simulink model "EKF2nd_order_4_parameters_simulink"  (R2022a)
settings: Solver=ode1  StartTime=0.0  StopTime=10  FixedStep=0.01  RelTol=1e-3
settings Model: Creator=Sarot PC  LastModifiedBy=LabPC
settings SolverCC: AlgebraicLoopSolver=TrustRegion
settings DebuggingCC: UnconnectedInputMsg=warning  UnconnectedOutputMsg=warning  UnconnectedLineMsg=warning  SFMachineParentedDataDiag=warning
settings RTWCC: DLArmComputeVersion=19.05

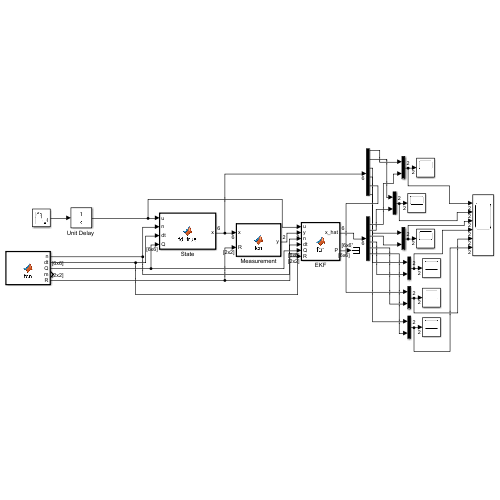
[thumbnail: Simulink's stored preview of the top-level diagram]
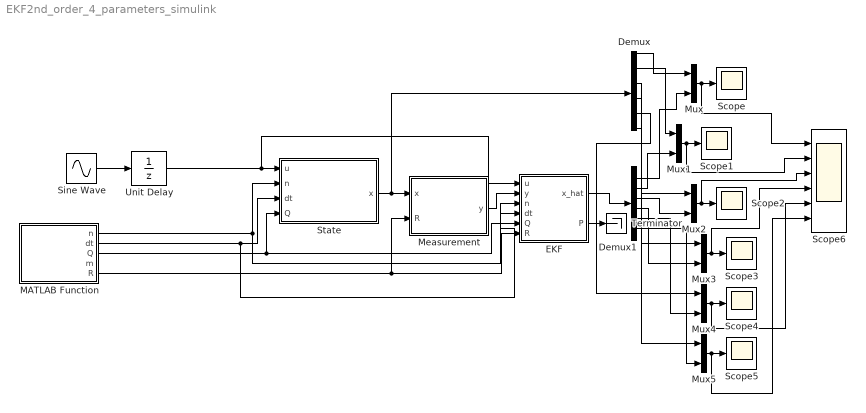
== system EKF2nd_order_4_parameters_simulink ==
  Demux : Demux  Outputs=6
  Demux1 : Demux  Outputs=6
  EKF : MATLAB Function  TreatAsAtomicUnit=on
  MATLAB Function : MATLAB Function  TreatAsAtomicUnit=on
  Measurement : MATLAB Function  TreatAsAtomicUnit=on
  Mux{,1..5} (6 alike) : Mux  Inputs=2
  Scope{,1..5} (6 alike) : Scope
  Scope6 : Scope  NumInputPorts=6
  Sine Wave : Sin  Amplitude=10  Frequency=2*pi*1.1
  State : MATLAB Function  TreatAsAtomicUnit=on
  Terminator : Terminator
  "Unit Delay " : UnitDelay  SampleTime=-1  HasFrameUpgradeWarning=on
  wires:
  State/1(x) -> Demux/1, Measurement/1(x)
  Measurement/1(y) -> EKF/2(y)
  EKF/1(x_hat) -> Demux1/1
  EKF/2(P) -> Terminator/1
  Demux/1 -> Mux/1
  Demux1/1 -> Mux/2
  Demux/2 -> Mux1/1
  Mux/1 -> Scope6/1, Scope/1
  Demux1/2 -> Mux1/2
  Demux/3 -> Mux2/1
  Demux1/3 -> Mux2/2
  Mux1/1 -> Scope6/2, Scope1/1
  Mux2/1 -> Scope6/3, Scope2/1
  Sine Wave/1 -> "Unit Delay "/1
  "Unit Delay "/1 -> EKF/1(u), State/1(u)
  MATLAB Function/1(n) -> EKF/3(n), State/2(n)
  MATLAB Function/2(dt) -> EKF/4(dt), State/3(dt)
  MATLAB Function/3(Q) -> EKF/5(Q), State/4(Q)
  MATLAB Function/5(R) -> EKF/6(R), Measurement/2(R)
  Mux3/1 -> Scope6/4, Scope3/1
  Demux/4 -> Mux3/1
  Demux1/4 -> Mux3/2
  Demux/5 -> Mux4/1
  Mux4/1 -> Scope6/5, Scope4/1
  Mux5/1 -> Scope6/6, Scope5/1
  Demux/6 -> Mux5/1
  Demux1/5 -> Mux4/2
  Demux1/6 -> Mux5/2

== matlab function EKF2nd_order_4_parameters_simulink/State ==
  settings: updateMethod=DISCRETE
  data: u input; x output; n input; dt input; Q input
function x = fd_true(u,n,dt,Q)

persistent x_
if isempty(x_),x_ = [0;0;10;20;40;30];end

% omega_ddot = -a*omega - b*omega_dot + c*u - d*sign(omega)
% Let x1=omega, x2=omega_dot, x3=a, x4=b, x5=c, x6=d
% x1_dot=-x2
% x2_dot=-x3*x1-x4*x2+x5*u-x6*sign(x1)
% x3_dot=0
% x4_dot=0
% x5_dot=0
% x6_dot=0

x = [x_(1) + dt*x_(2)
     x_(2) + dt*(-x_(3)*x_(1) - x_(4)*x_(2) + x_(5)*u - x_(6)*sign(x_(1)))
     x_(3)
     x_(4)
     x_(5)
     x_(6)] + sqrt(dt)*sqrt(Q)*randn(n,1);
x_= x;

== matlab function EKF2nd_order_4_parameters_simulink/MATLAB Function ==
  data: n output; dt output; Q output; m output; R output
function [n,dt,Q,m,R] = fcn

n  = 6;
m  = 2;
dt = 0.01;

Q = 1e-6*diag([0 1 1 1 1 1]);
R = 1e-3*diag([1 10]);

== matlab function EKF2nd_order_4_parameters_simulink/Measurement ==
  data: x input; y output; R input
function y = fcn(x,R)


C = [1 0 0 0 0 0
     0 1 0 0 0 0];

y = C*x+sqrt(R)*randn(2,1);

== matlab function EKF2nd_order_4_parameters_simulink/EKF ==
  settings: updateMethod=DISCRETE
  data: u input; x_hat output; P output; y input; n input; dt input; Q input; R input
function [x_hat,P] = fcn(u,y,n,dt,Q,R)

persistent x_ P_
if isempty(x_), x_= randn(n,1); P_ = 1e0*eye(n); end


x = x_ + dt*[ x_(2)
             -x_(3)*x_(1)-x_(4)*x_(2)+x_(5)*u-x_(6)*sign(x_(1))
              0
              0
              0
              0];
 

A = eye(6) + dt*[0      1       0       0       0       0
                -x_(3) -x_(4)  -x_(1)  -x_(2)   u     -sign(x_(1))
                 0      0       0       0       0       0
                 0      0       0       0       0       0
                 0      0       0       0       0       0
                 0      0       0       0       0       0];
x_hat = x;

C = [1 0 0 0 0 0
     0 1 0 0 0 0];
P = A*P_*A'+ Q + 1e-4*diag([0 0 1000 10 10 1000]);

W = (P*C')/(C*P*C'+ 1*R);
x_ = x + W*(y-C*x);
P_ = P - W*C*P;
